simulink subsystem "sensor_baro"  (R2026a)
settings: Solver=VariableStepAuto
model mask{samplingrate=100, noise_pres=0.2, bias_pres=0, scale_pres=1, limit_pres=[0, inf]}
  mask prompts: samplingrate "Sampling Time (s)"; noise_pres "Pressure Noise Power"; bias_pres "Pressure Bias"; scale_pres "Pressure Scaling"; limit_pres "Pressure Limit"
libraries: simulink x1, aerolibatmos2 x1
settings Model: Creator=finnb  LastModifiedBy=trist

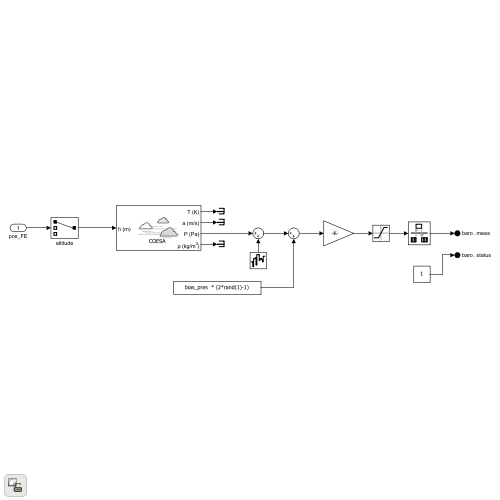
[thumbnail: Simulink's stored preview of the top-level diagram]
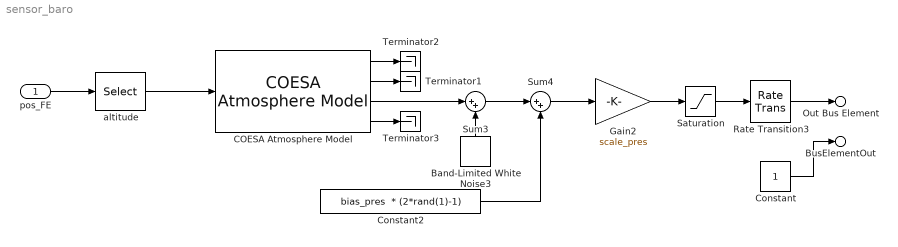
== system sensor_baro ==
  pos_FE : Inport
  Band-Limited White Noise3 : simulink/Sources/Band-Limited White Noise  Cov=noise_pres  Ts=samplingrate  seed=[5781]
  COESA Atmosphere Model : aerolibatmos2/COESA Atmosphere Model  units=Metric (MKS)  spec=1976 COESA-extended U.S. Standard Atmosphere  model=Profile  profile_var=High temperature  profile_percent=1%  profile_alt=5 km (16404 ft)  envelope_var=High temperature  envelope_percent=1%  action=Warning
  Constant : Constant  OutDataTypeStr=boolean
  Constant2 : Constant  Value="bias_pres  * (2*rand(1)-1)"
  Gain2 : Gain  Gain=scale_pres
  Rate Transition3 : RateTransition  OutPortSampleTime=samplingrate
  Saturation : Saturate  UpperLimit=limit_pres(2)  LowerLimit=limit_pres(1)
  Sum3 : Sum  Inputs=|++
  Sum4 : Sum  Inputs=|++
  Terminator1 : Terminator
  Terminator2 : Terminator
  Terminator3 : Terminator
  altitude : Selector  InputPortWidth=3  IndexOptions=Index vector (dialog)  Indices=[1]  OutputSizes=1
  Out Bus Element : Outport  PortName=baro  Element=meas
  BusElementOut : Outport  PortName=baro  Element=status
  wires:
  Sum3/1 -> Sum4/1
  Band-Limited White Noise3/1 -> Sum3/2
  pos_FE/1 -> altitude/1
  Sum4/1 -> Gain2/1
  Constant2/1 -> Sum4/2
  Gain2/1 -> Saturation/1
  Saturation/1 -> Rate Transition3/1
  Rate Transition3/1 -> Out Bus Element/1
  Constant/1 -> BusElementOut/1
  COESA Atmosphere Model/2 -> Terminator1/1
  COESA Atmosphere Model/3 -> Sum3/1
  COESA Atmosphere Model/4 -> Terminator3/1
  altitude/1 -> COESA Atmosphere Model/1
  COESA Atmosphere Model/1 -> Terminator2/1
